simulink model "G431Hallcorrection"  (R2024a)
settings: Solver=FixedStepAuto  StartTime=0.0  StopTime=inf  RelTol=1e-3  EnableMultiTasking=on
undefined symbols (not defined in the file): DiscIntNeverNeededParam
libraries: stm32f4xxblockslib x11, mcbcontrolslib x7, simulink x6, mcbpositiondecoderlib x4, stm32g4xxblockslib x3, stm32blockslib x3, mcbsensorlessestimatorlib x2
settings Model: Creator=wsl  LastModifiedBy=wsl
settings SolverCC: AutoInsertRateTranBlk=on
settings DataIOCC: ReturnWorkspaceOutputs=off
settings OptimizationCC: EnhancedBackFolding=on  PassReuseOutputArgsAs=Individual arguments  ZeroExternalMemoryAtStartup=off  ZeroInternalMemoryAtStartup=off  MaxStackSize=64  OptimizeBlockOrder=speed  DifferentSizesBufferReuse=on  OptimizationCustomize=off  EfficientTunableParamExpr=on
settings DebuggingCC: MultiTaskDSMMsg=none  TasksWithSamePriorityMsg=none  ParameterPrecisionLossMsg=none  ParameterTunabilityLossMsg=error
settings HardwareCC: ProdBitPerPointer=32  ProdBitPerSizeT=32  ProdBitPerPtrDiffT=32  ProdLargestAtomicInteger=Long  ProdLargestAtomicFloat=Double  ProdWordSize=32  ProdLongLongMode=on  ProdHWDeviceType=ARM Compatible->ARM Cortex-M
settings SFSimCC: MATLABDynamicMemAlloc=off
settings RTWCC: Description=Embedded Coder  SystemTargetFile=ert.tlc  HardwareBoard=STM32G4xx Based  TemplateMakefile=ert_default_tmf  Toolchain=GNU Tools for ARM Embedded Processors
settings CodeAppCC: ForceParamTrailComments=on  IgnoreCustomStorageClasses=off  OperatorAnnotations=on  SimulinkDataObjDesc=on  SFDataObjDesc=on  InsertBlockDesc=on
settings ERTTargetCC: TargetLangStandard=C99 (ISO)  CodeReplacementLibrary=ARM Cortex-M  ExtModeTransport=3  ExtModeStaticAlloc=on  ExtModeStaticAllocSize=2048  ExtModeMexFile=ext_xcp  ExtModeIntrfLevel=Level2 - Open

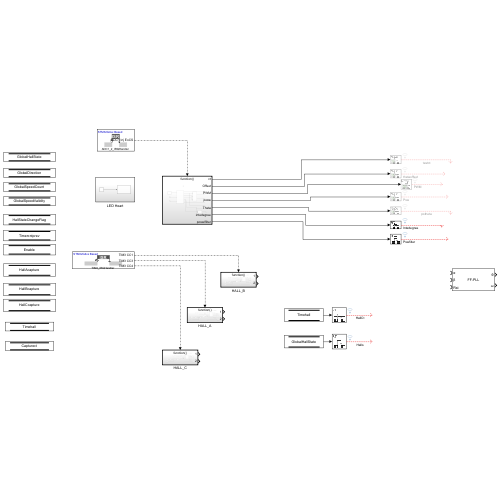
[thumbnail: Simulink's stored preview of the top-level diagram]
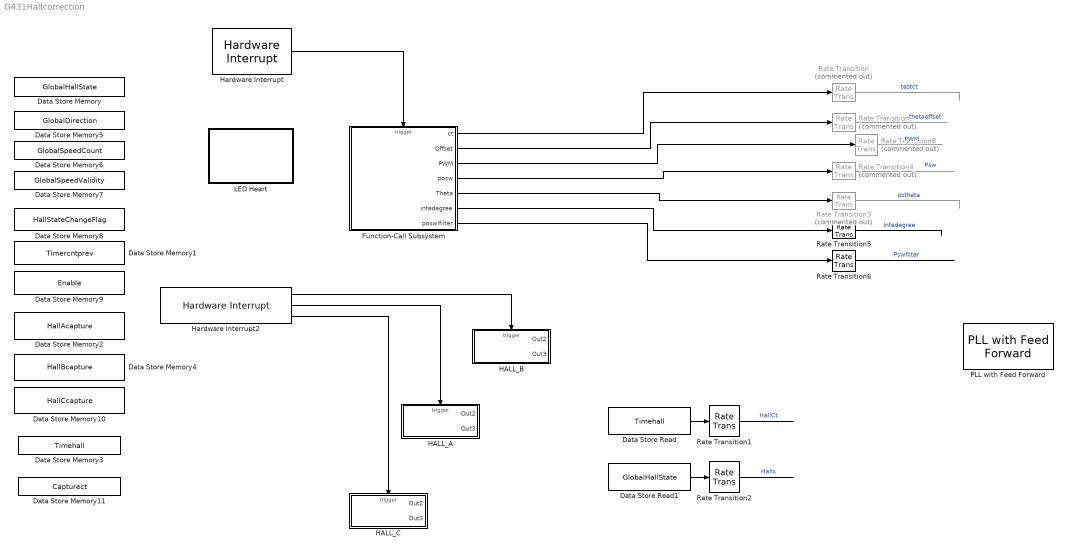
== system G431Hallcorrection ==
  Data Store Memory : DataStoreMemory  DataStoreName=GlobalHallState  WriteAfterWriteMsg=warning  ShowAdditionalParam=off
  Data Store Memory1 : DataStoreMemory  DataStoreName=Timercntprev  WriteAfterWriteMsg=warning  ShowAdditionalParam=off
  Data Store Memory10 : DataStoreMemory  DataStoreName=HallCcapture  WriteAfterWriteMsg=warning  ShowAdditionalParam=off
  Data Store Memory11 : DataStoreMemory  DataStoreName=Capturect  WriteAfterWriteMsg=warning  ShowAdditionalParam=off
  Data Store Memory2 : DataStoreMemory  DataStoreName=HallAcapture  WriteAfterWriteMsg=warning  ShowAdditionalParam=off
  Data Store Memory3 : DataStoreMemory  DataStoreName=Timehall  WriteAfterWriteMsg=warning  ShowAdditionalParam=off
  Data Store Memory4 : DataStoreMemory  DataStoreName=HallBcapture  WriteAfterWriteMsg=warning  ShowAdditionalParam=off
  Data Store Memory5 : DataStoreMemory  DataStoreName=GlobalDirection  WriteAfterWriteMsg=warning  ShowAdditionalParam=off
  Data Store Memory6 : DataStoreMemory  DataStoreName=GlobalSpeedCount  WriteAfterWriteMsg=warning  ShowAdditionalParam=off
  Data Store Memory7 : DataStoreMemory  DataStoreName=GlobalSpeedValidity  WriteAfterWriteMsg=warning  ShowAdditionalParam=off
  Data Store Memory8 : DataStoreMemory  DataStoreName=HallStateChangeFlag  WriteAfterWriteMsg=warning  ShowAdditionalParam=off
  Data Store Memory9 : DataStoreMemory  DataStoreName=Enable  WriteAfterWriteMsg=warning  ShowAdditionalParam=off
  Data Store Read : DataStoreRead  DataStoreName=Timehall  IndexOptions=Index vector (dialog)  Indices=1  OutputSizes=1
  Data Store Read1 : DataStoreRead  DataStoreName=GlobalHallState  IndexOptions=Index vector (dialog)  Indices=1  OutputSizes=1
  Function-Call Subsystem : Subsystem  TreatAsAtomicUnit=on
  HALL_A : Subsystem  TreatAsAtomicUnit=on
  HALL_B : Subsystem  TreatAsAtomicUnit=on
  HALL_C : Subsystem  TreatAsAtomicUnit=on
  Hardware Interrupt : stm32g4xxblockslib/Hardware Interrupt  ISRGroup=Analog to digital converter (ADC)  ISRName=ADC1_2_IRQHandler  ISRNumber=33  EventsList={ 'off', 'ADC1 OVR', '1'; 'off', 'ADC1 Reg EoCS', '2'; 'on', 'ADC1 Inj EoCS', '3'; 'off', 'ADC1 Inj JQOVF', '4'; 'off', 'ADC1 Watchdog1', '5'; 'off', 'ADC1 Watchdog2', '6'; 'off', 'ADC1 Watchdog3', '7'; 'off', 'ADC2 OVR', '8'; 'off', 'ADC2 Reg EoCS', '9'; 'off', 'ADC2 Inj EoCS', '10'; 'off', 'ADC2 Inj JQOVF', '11'; 'off', 'ADC2 Watchdog', '12'; 'off', 'ADC2 Watchdog2', '13'; 'off', 'ADC2 Watchdog3', '14'; 'off', 'Custom event', '15' }  SelectedEvents={'ADC1 Inj EoCS'}  TaskPriority=30  DisablePreemption=on  ClearInterruptFlagsAtEndOfEvent=off  InterruptDefinitionFile=$(TARGET_ROOT)/registry/interrupts/STM32F4xxBased_interrupts.xml  HardwareBoard=STM32G4xx Based  EnableSimPort=off
  Hardware Interrupt2 : stm32g4xxblockslib/Hardware Interrupt  ISRGroup=Timer (TIM)  ISRName=TIM3_IRQHandler  ISRNumber=44  EventsList={ 'off', 'TIM3 Update', '1'; 'on', 'TIM3 CC1', '2'; 'off', 'TIM3 CC2', '3'; 'on', 'TIM3 CC3', '4'; 'on', 'TIM3 CC4', '5'; 'off', 'TIM3 Trigger', '6'; 'off', 'TIM3 DIR', '7'; 'off', 'TIM3 IDX', '8'; 'off', 'TIM3 IERR', '9'; 'off', 'TIM3 TERR', '10'; 'off', 'Custom event', '11' }  SelectedEvents={'TIM3 CC1','TIM3 CC3','TIM3 CC4'}  TaskPriority=29  DisablePreemption=on  ClearInterruptFlagsAtEndOfEvent=off  InterruptDefinitionFile=$(TARGET_ROOT)/registry/interrupts/STM32F4xxBased_interrupts.xml  HardwareBoard=STM32G4xx Based  EnableSimPort=off
  LED Heart : Subsystem
  PLL with Feed Forward : mcbsensorlessestimatorlib/PLL with Feed Forward  Normalization=on  PosOut=Angular position  BlkSampleTime=50e-6  FreqRatio=1  MaximumApplicationFreq=7500  SpeedCutoffFreq=15  N_points=1024  Kp=942.4778  Ki=222066.099  PositionUnit=Degrees  PositionDataType=single  FrequencyUnit=Degrees/Sec  FrequencyDataType=single  TableDataType=single
      settings: LibrarySourceBlock=mcblib/Signal Management/PLL with Feed Forward
  Rate Transition{,3..4,7..8} (5 alike) : RateTransition  Commented=on  Integrity=off  OutPortSampleTime=1e-3
  Rate Transition{1..2,5..6} (4 alike) : RateTransition  Integrity=off  OutPortSampleTime=1e-3
  wires:
  Hardware Interrupt/1 -> Function-Call Subsystem/Trigger
  Function-Call Subsystem/1(ct) -> Rate Transition/1
  Rate Transition/1 -> ?  "testct"
  Data Store Read/1 -> Rate Transition1/1
  Rate Transition1/1 -> ?  "HallCt"
  Hardware Interrupt2/3 -> HALL_C/Trigger
  Hardware Interrupt2/1 -> HALL_B/Trigger
  Hardware Interrupt2/2 -> HALL_A/Trigger
  Rate Transition2/1 -> ?  "Halls"
  Data Store Read1/1 -> Rate Transition2/1
  Rate Transition3/1 -> ?  "pstheta"
  Function-Call Subsystem/5(Theta) -> Rate Transition3/1
  Rate Transition4/1 -> ?  "Psw"
  Function-Call Subsystem/6(intedegree) -> Rate Transition5/1
  Rate Transition5/1 -> ?  "Intedegree"
  Function-Call Subsystem/4(posw) -> Rate Transition4/1
  Rate Transition6/1 -> ?  "Pswfilter"
  Function-Call Subsystem/7(poswlfilter) -> Rate Transition6/1
  Function-Call Subsystem/2(Offset) -> Rate Transition7/1
  Rate Transition7/1 -> ?  "thetaoffset"
  Function-Call Subsystem/3(PWM) -> Rate Transition8/1
  Rate Transition8/1 -> ?  "PWM"

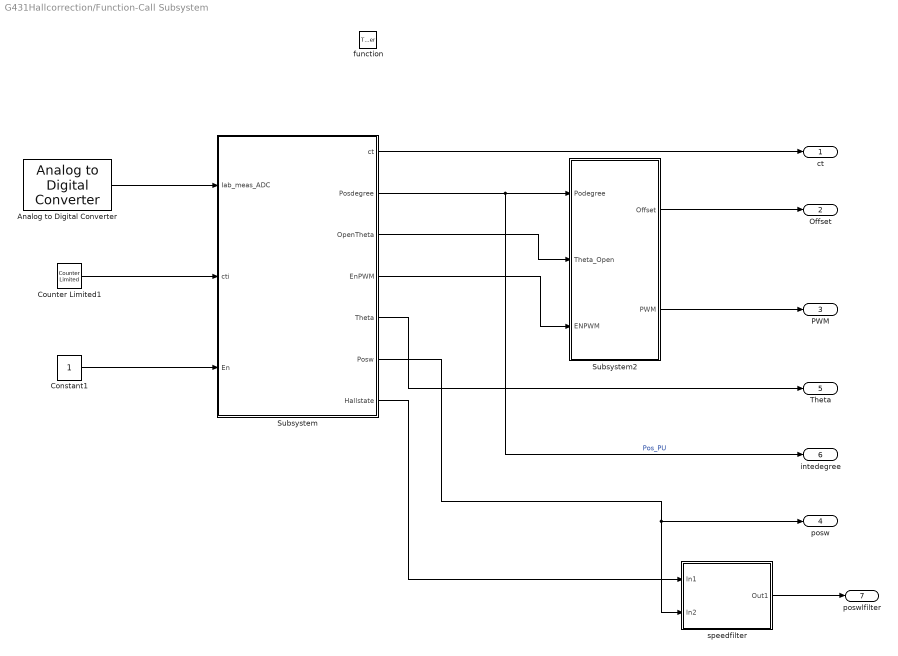
== system G431Hallcorrection/Function-Call Subsystem ==
  function : TriggerPort  TriggerType=function-call  VariantControl=(inherit)
  Analog to Digital Converter : stm32f4xxblockslib/Analog to Digital Converter  ADCModule=ADC1  ConversionGroup=Injected  TriggerMode=Read results only  NumberOfConversions=3  EnableBufferConv=off  BufferLength=1  OutputStatus=off  SampleTime=-1  EnableSimPort=off
  Constant1 : Constant  VectorParams1D=off
  Counter Limited1 : simulink/Sources/Counter Limited  uplimit=20000  tsamp=-1
  Subsystem : Subsystem
  Subsystem2 : Subsystem
  "speedfilter " : Subsystem
  ct : Outport
  Offset : Outport  Port=2
  PWM : Outport  Port=3
  posw : Outport  Port=4
  Theta : Outport  Port=5
  intedegree : Outport  Port=6
  poswlfilter : Outport  Port=7
  wires:
  Analog to Digital Converter/1 -> Subsystem/1(Iab_meas_ADC)
  Subsystem/4(EnPWM) -> Subsystem2/3(ENPWM)
  Subsystem2/2(PWM) -> PWM/1
  Constant1/1 -> Subsystem/3(En)
  Subsystem/1(ct) -> ct/1
  Subsystem2/1(Offset) -> Offset/1
  Subsystem/2(Posdegree) -> intedegree/1, Subsystem2/1(Podegree)  "Pos_PU"
  Counter Limited1/1 -> Subsystem/2(cti)
  Subsystem/3(OpenTheta) -> Subsystem2/2(Theta_Open)
  Subsystem/5(Theta) -> Theta/1
  Subsystem/6(Posw) -> "speedfilter "/2(In2), posw/1
  Subsystem/7(Hallstate) -> "speedfilter "/1(In1)
  "speedfilter "/1(Out1) -> poswlfilter/1

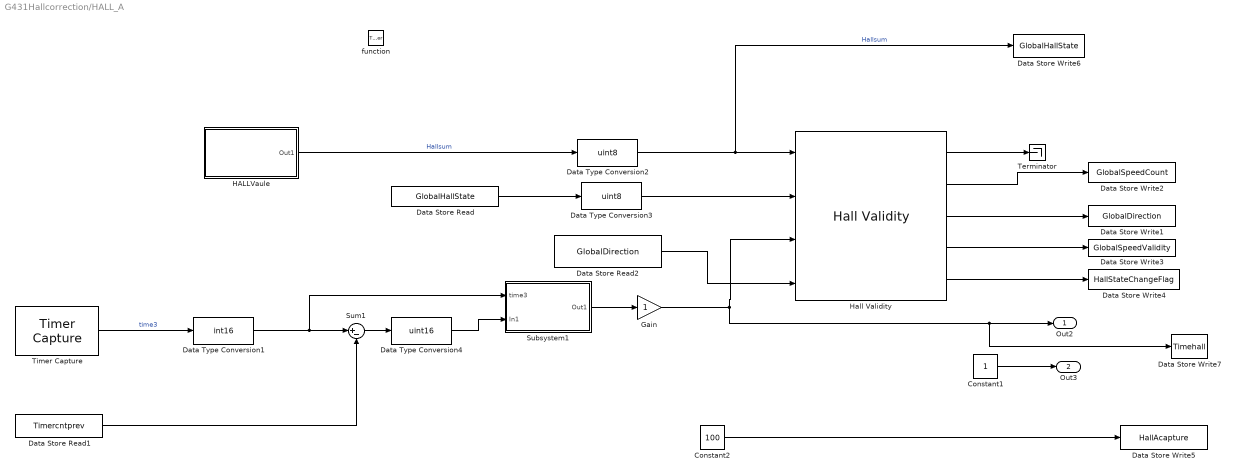
== system G431Hallcorrection/HALL_A ==
  function : TriggerPort  TriggerType=function-call  VariantControl=(inherit)
  Constant1 : Constant
  Constant2 : Constant  Value=100
  Data Store Read : DataStoreRead  DataStoreName=GlobalHallState  IndexOptions=Index vector (dialog)  Indices=1  OutputSizes=1
  Data Store Read1 : DataStoreRead  DataStoreName=Timercntprev  IndexOptions=Index vector (dialog)  Indices=1  OutputSizes=1
  Data Store Read2 : DataStoreRead  DataStoreName=GlobalDirection  IndexOptions=Index vector (dialog)  Indices=1  OutputSizes=1
  Data Store Write1 : DataStoreWrite  DataStoreName=GlobalDirection  IndexOptions=Index vector (dialog)  Indices=1  OutputSizes=1
  Data Store Write2 : DataStoreWrite  DataStoreName=GlobalSpeedCount  IndexOptions=Index vector (dialog)  Indices=1  OutputSizes=1
  Data Store Write3 : DataStoreWrite  DataStoreName=GlobalSpeedValidity  IndexOptions=Index vector (dialog)  Indices=1  OutputSizes=1
  Data Store Write4 : DataStoreWrite  DataStoreName=HallStateChangeFlag  IndexOptions=Index vector (dialog)  Indices=1  OutputSizes=1
  Data Store Write5 : DataStoreWrite  DataStoreName=HallAcapture  IndexOptions=Index vector (dialog)  Indices=1  OutputSizes=1
  Data Store Write6 : DataStoreWrite  DataStoreName=GlobalHallState  IndexOptions=Index vector (dialog)  Indices=1  OutputSizes=1
  Data Store Write7 : DataStoreWrite  DataStoreName=Timehall  IndexOptions=Index vector (dialog)  Indices=1  OutputSizes=1
  Data Type Conversion1 : DataTypeConversion  OutDataTypeStr=int16  SaturateOnIntegerOverflow=off  RndMeth=Floor
  Data Type Conversion2 : DataTypeConversion  OutDataTypeStr=uint8  SaturateOnIntegerOverflow=off  RndMeth=Floor
  Data Type Conversion3 : DataTypeConversion  OutDataTypeStr=uint8  SaturateOnIntegerOverflow=off  RndMeth=Floor
  Data Type Conversion4 : DataTypeConversion  OutDataTypeStr=uint16  SaturateOnIntegerOverflow=off  RndMeth=Floor
  Gain : Gain
  HALLVaule : Subsystem
  Hall Validity : mcbpositiondecoderlib/Hall Validity  hallSequence=ABC  sequence=[5,4,6,2,3,1]  CounterSize=16 bits
  Subsystem1 : Subsystem
  Sum1 : Sum  Inputs=|+-
  Terminator : Terminator
  Timer Capture : stm32blockslib/Timer Capture  TimerModule=TIM3  SelectedChannel=CH3  CaptureLength=1  OutputDataLength=off  OutputOverrunStatus=off  OutputDirection=off  SampleTime=-1
      settings: LibrarySourceBlock=stm32g4xxblockslib/Timer Capture
  Out2 : Outport
  Out3 : Outport  Port=2
  wires:
  Hall Validity/4 -> Data Store Write3/1
  HALLVaule/1(Out1) -> Data Type Conversion2/1  "Hallsum"
  Data Type Conversion3/1 -> Hall Validity/2
  Data Store Read2/1 -> Hall Validity/4
  Gain/1 -> Data Store Write7/1, Out2/1, Hall Validity/3
  Data Type Conversion2/1 -> Data Store Write6/1, Hall Validity/1  "Hallsum"
  Hall Validity/3 -> Data Store Write1/1
  Constant1/1 -> Out3/1
  Hall Validity/2 -> Data Store Write2/1
  Hall Validity/1 -> Terminator/1
  Constant2/1 -> Data Store Write5/1
  Hall Validity/5 -> Data Store Write4/1
  Data Store Read/1 -> Data Type Conversion3/1
  Sum1/1 -> Data Type Conversion4/1
  Data Store Read1/1 -> Sum1/2
  Data Type Conversion1/1 -> Sum1/1, Subsystem1/1(time3)
  Timer Capture/1 -> Data Type Conversion1/1  "time3"
  Data Type Conversion4/1 -> Subsystem1/2(In1)
  Subsystem1/1(Out1) -> Gain/1

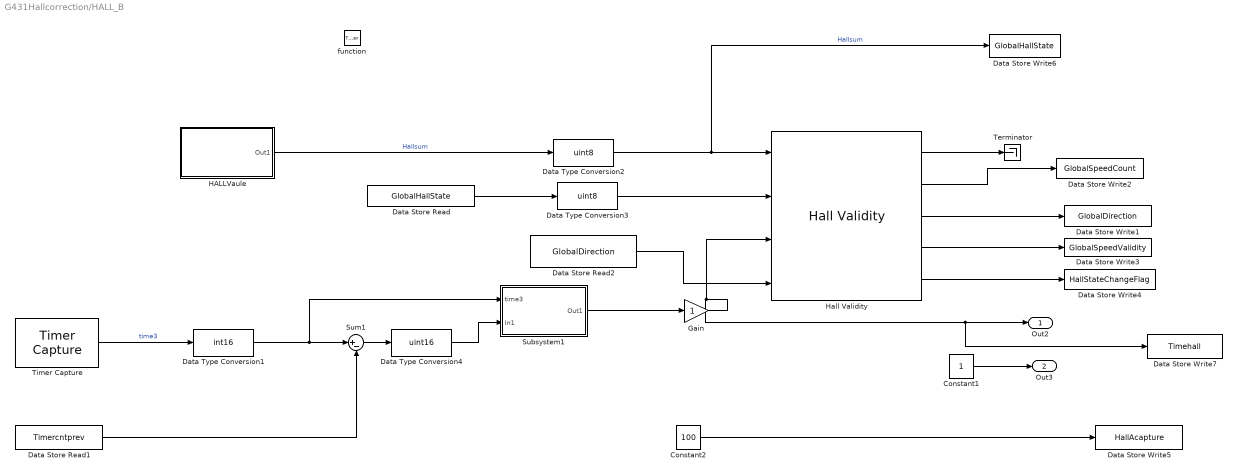
== system G431Hallcorrection/HALL_B ==
  function : TriggerPort  TriggerType=function-call  VariantControl=(inherit)
  Constant1 : Constant
  Constant2 : Constant  Value=100
  Data Store Read : DataStoreRead  DataStoreName=GlobalHallState  IndexOptions=Index vector (dialog)  Indices=1  OutputSizes=1
  Data Store Read1 : DataStoreRead  DataStoreName=Timercntprev  IndexOptions=Index vector (dialog)  Indices=1  OutputSizes=1
  Data Store Read2 : DataStoreRead  DataStoreName=GlobalDirection  IndexOptions=Index vector (dialog)  Indices=1  OutputSizes=1
  Data Store Write1 : DataStoreWrite  DataStoreName=GlobalDirection  IndexOptions=Index vector (dialog)  Indices=1  OutputSizes=1
  Data Store Write2 : DataStoreWrite  DataStoreName=GlobalSpeedCount  IndexOptions=Index vector (dialog)  Indices=1  OutputSizes=1
  Data Store Write3 : DataStoreWrite  DataStoreName=GlobalSpeedValidity  IndexOptions=Index vector (dialog)  Indices=1  OutputSizes=1
  Data Store Write4 : DataStoreWrite  DataStoreName=HallStateChangeFlag  IndexOptions=Index vector (dialog)  Indices=1  OutputSizes=1
  Data Store Write5 : DataStoreWrite  DataStoreName=HallAcapture  IndexOptions=Index vector (dialog)  Indices=1  OutputSizes=1
  Data Store Write6 : DataStoreWrite  DataStoreName=GlobalHallState  IndexOptions=Index vector (dialog)  Indices=1  OutputSizes=1
  Data Store Write7 : DataStoreWrite  DataStoreName=Timehall  IndexOptions=Index vector (dialog)  Indices=1  OutputSizes=1
  Data Type Conversion1 : DataTypeConversion  OutDataTypeStr=int16  SaturateOnIntegerOverflow=off  RndMeth=Floor
  Data Type Conversion2 : DataTypeConversion  OutDataTypeStr=uint8  SaturateOnIntegerOverflow=off  RndMeth=Floor
  Data Type Conversion3 : DataTypeConversion  OutDataTypeStr=uint8  SaturateOnIntegerOverflow=off  RndMeth=Floor
  Data Type Conversion4 : DataTypeConversion  OutDataTypeStr=uint16  SaturateOnIntegerOverflow=off  RndMeth=Floor
  Gain : Gain
  HALLVaule : Subsystem
  Hall Validity : mcbpositiondecoderlib/Hall Validity  hallSequence=ABC  sequence=[5,4,6,2,3,1]  CounterSize=16 bits
  Subsystem1 : Subsystem
  Sum1 : Sum  Inputs=|+-
  Terminator : Terminator
  Timer Capture : stm32blockslib/Timer Capture  TimerModule=TIM3  SelectedChannel=CH1  CaptureLength=1  OutputDataLength=off  OutputOverrunStatus=off  OutputDirection=off  SampleTime=-1
      settings: LibrarySourceBlock=stm32g4xxblockslib/Timer Capture
  Out2 : Outport
  Out3 : Outport  Port=2
  wires:
  Hall Validity/4 -> Data Store Write3/1
  HALLVaule/1(Out1) -> Data Type Conversion2/1  "Hallsum"
  Data Type Conversion3/1 -> Hall Validity/2
  Data Store Read2/1 -> Hall Validity/4
  Gain/1 -> Data Store Write7/1, Out2/1, Hall Validity/3
  Data Type Conversion2/1 -> Data Store Write6/1, Hall Validity/1  "Hallsum"
  Hall Validity/3 -> Data Store Write1/1
  Constant1/1 -> Out3/1
  Hall Validity/1 -> Terminator/1
  Constant2/1 -> Data Store Write5/1
  Hall Validity/5 -> Data Store Write4/1
  Data Store Read/1 -> Data Type Conversion3/1
  Data Type Conversion4/1 -> Subsystem1/2(In1)
  Sum1/1 -> Data Type Conversion4/1
  Timer Capture/1 -> Data Type Conversion1/1  "time3"
  Data Type Conversion1/1 -> Sum1/1, Subsystem1/1(time3)
  Data Store Read1/1 -> Sum1/2
  Subsystem1/1(Out1) -> Gain/1
  Hall Validity/2 -> Data Store Write2/1

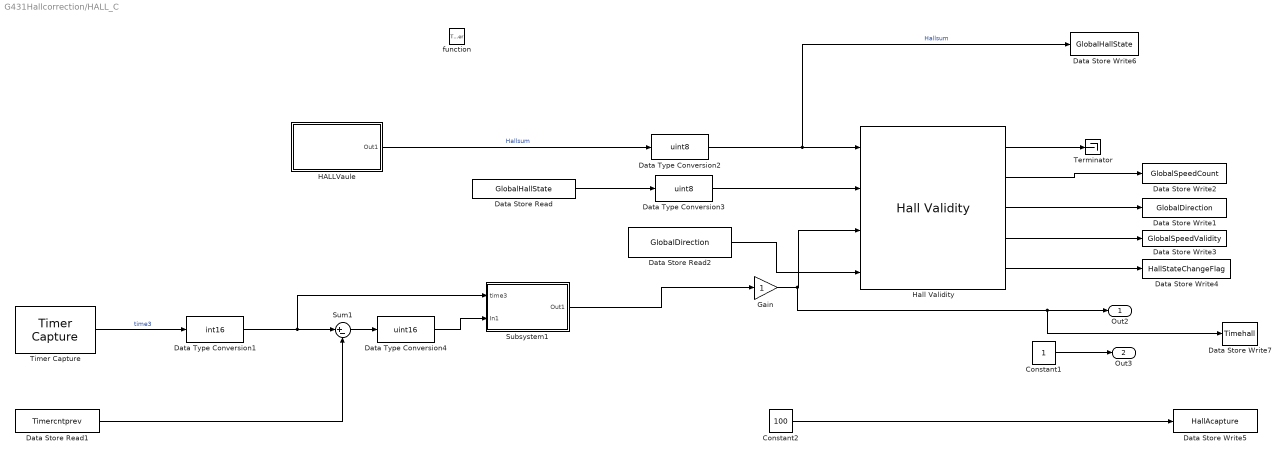
== system G431Hallcorrection/HALL_C ==
  function : TriggerPort  TriggerType=function-call  VariantControl=(inherit)
  Constant1 : Constant
  Constant2 : Constant  Value=100
  Data Store Read : DataStoreRead  DataStoreName=GlobalHallState  IndexOptions=Index vector (dialog)  Indices=1  OutputSizes=1
  Data Store Read1 : DataStoreRead  DataStoreName=Timercntprev  IndexOptions=Index vector (dialog)  Indices=1  OutputSizes=1
  Data Store Read2 : DataStoreRead  DataStoreName=GlobalDirection  IndexOptions=Index vector (dialog)  Indices=1  OutputSizes=1
  Data Store Write1 : DataStoreWrite  DataStoreName=GlobalDirection  IndexOptions=Index vector (dialog)  Indices=1  OutputSizes=1
  Data Store Write2 : DataStoreWrite  DataStoreName=GlobalSpeedCount  IndexOptions=Index vector (dialog)  Indices=1  OutputSizes=1
  Data Store Write3 : DataStoreWrite  DataStoreName=GlobalSpeedValidity  IndexOptions=Index vector (dialog)  Indices=1  OutputSizes=1
  Data Store Write4 : DataStoreWrite  DataStoreName=HallStateChangeFlag  IndexOptions=Index vector (dialog)  Indices=1  OutputSizes=1
  Data Store Write5 : DataStoreWrite  DataStoreName=HallAcapture  IndexOptions=Index vector (dialog)  Indices=1  OutputSizes=1
  Data Store Write6 : DataStoreWrite  DataStoreName=GlobalHallState  IndexOptions=Index vector (dialog)  Indices=1  OutputSizes=1
  Data Store Write7 : DataStoreWrite  DataStoreName=Timehall  IndexOptions=Index vector (dialog)  Indices=1  OutputSizes=1
  Data Type Conversion1 : DataTypeConversion  OutDataTypeStr=int16  SaturateOnIntegerOverflow=off  RndMeth=Floor
  Data Type Conversion2 : DataTypeConversion  OutDataTypeStr=uint8  SaturateOnIntegerOverflow=off  RndMeth=Floor
  Data Type Conversion3 : DataTypeConversion  OutDataTypeStr=uint8  SaturateOnIntegerOverflow=off  RndMeth=Floor
  Data Type Conversion4 : DataTypeConversion  OutDataTypeStr=uint16  SaturateOnIntegerOverflow=off  RndMeth=Floor
  Gain : Gain
  HALLVaule : Subsystem
  Hall Validity : mcbpositiondecoderlib/Hall Validity  hallSequence=ABC  sequence=[5,4,6,2,3,1]  CounterSize=16 bits
  Subsystem1 : Subsystem
  Sum1 : Sum  Inputs=|+-
  Terminator : Terminator
  Timer Capture : stm32blockslib/Timer Capture  TimerModule=TIM3  SelectedChannel=CH4  CaptureLength=1  OutputDataLength=off  OutputOverrunStatus=off  OutputDirection=off  SampleTime=-1
      settings: LibrarySourceBlock=stm32g4xxblockslib/Timer Capture
  Out2 : Outport
  Out3 : Outport  Port=2
  wires:
  Hall Validity/4 -> Data Store Write3/1
  HALLVaule/1(Out1) -> Data Type Conversion2/1  "Hallsum"
  Data Type Conversion3/1 -> Hall Validity/2
  Data Store Read2/1 -> Hall Validity/4
  Gain/1 -> Data Store Write7/1, Out2/1, Hall Validity/3
  Data Type Conversion2/1 -> Data Store Write6/1, Hall Validity/1  "Hallsum"
  Hall Validity/3 -> Data Store Write1/1
  Constant1/1 -> Out3/1
  Hall Validity/1 -> Terminator/1
  Constant2/1 -> Data Store Write5/1
  Hall Validity/5 -> Data Store Write4/1
  Data Store Read/1 -> Data Type Conversion3/1
  Data Type Conversion4/1 -> Subsystem1/2(In1)
  Sum1/1 -> Data Type Conversion4/1
  Timer Capture/1 -> Data Type Conversion1/1  "time3"
  Data Type Conversion1/1 -> Sum1/1, Subsystem1/1(time3)
  Data Store Read1/1 -> Sum1/2
  Subsystem1/1(Out1) -> Gain/1
  Hall Validity/2 -> Data Store Write2/1

== system G431Hallcorrection/LED Heart ==
  Digital Port Write : stm32f4xxblockslib/Digital Port Write  PortName=GPIOA  PinNumber=[5]  ReadOperation=off  IOAsArray=on  EnableSimPort=off
      settings: LibrarySourceBlock=stm32g4xxblockslib/Digital Port Write
  Pulse Generator : DiscretePulseGenerator  Period=10  PulseWidth=5  SampleTime=0.1
  wires:
  Pulse Generator/1 -> Digital Port Write/1  "LED"

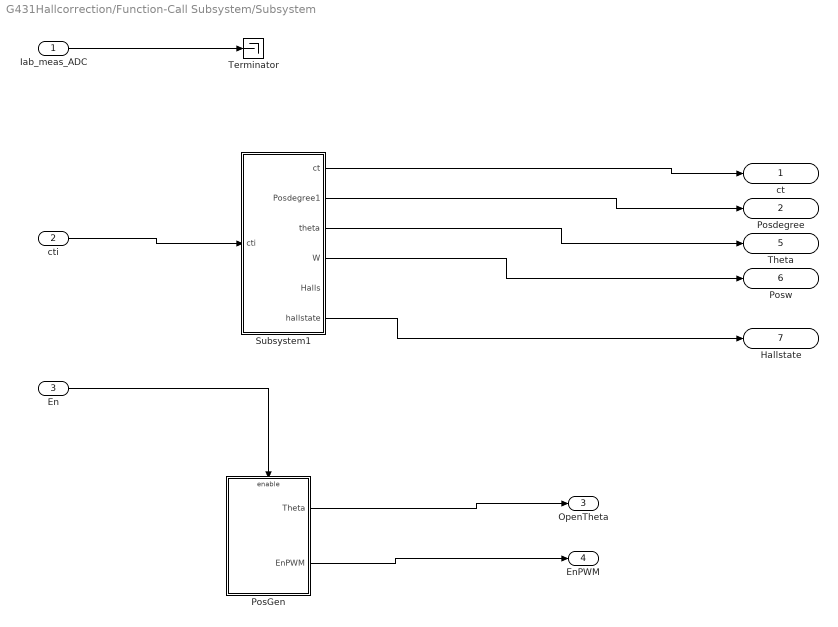
== system G431Hallcorrection/Function-Call Subsystem/Subsystem ==
  Iab_meas_ADC : Inport  OutDataTypeStr=uint16
  cti : Inport  Port=2
  En : Inport  Port=3
  PosGen : Subsystem
  Subsystem1 : Subsystem
  Terminator : Terminator
  ct : Outport
  Posdegree : Outport  Port=2
  OpenTheta : Outport  Port=3
  EnPWM : Outport  Port=4
  Theta : Outport  Port=5
  Posw : Outport  Port=6
  Hallstate : Outport  Port=7
  wires:
  Iab_meas_ADC/1 -> Terminator/1
  Subsystem1/2(Posdegree1) -> Posdegree/1
  Subsystem1/1(ct) -> ct/1
  cti/1 -> Subsystem1/1(cti)
  PosGen/1(Theta) -> OpenTheta/1
  PosGen/2(EnPWM) -> EnPWM/1
  En/1 -> PosGen/Enable
  Subsystem1/3(theta) -> Theta/1
  Subsystem1/4(W) -> Posw/1
  Subsystem1/6(hallstate) -> Hallstate/1

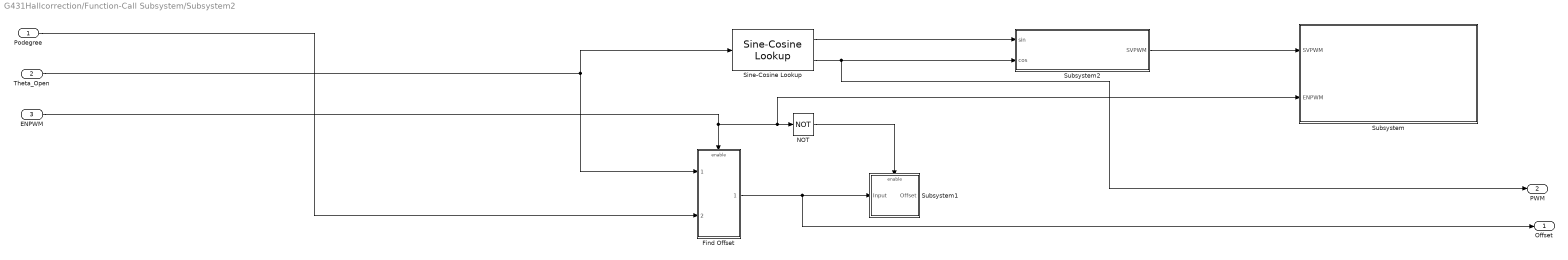
== system G431Hallcorrection/Function-Call Subsystem/Subsystem2 ==
  Podegree : Inport
  Theta_Open : Inport  Port=2
  ENPWM : Inport  Port=3
  Find Offset : Subsystem
  NOT : Logic  Operator=NOT  IconShape=distinctive  AllPortsSameDT=off  OutDataTypeStr=boolean
  Sine-Cosine Lookup : mcbcontrolslib/Sine-Cosine Lookup  AngleInput=Per-unit  N_points=1024  DatatypeInput=Inherit from input  Datatype=single
  Subsystem : Subsystem
  Subsystem1 : Subsystem
  Subsystem2 : Subsystem
  Offset : Outport
  PWM : Outport  Port=2
  wires:
  ENPWM/1 -> Subsystem/2(ENPWM), NOT/1, Find Offset/Enable
  Podegree/1 -> Find Offset/2(Theta_hall)
  Theta_Open/1 -> Sine-Cosine Lookup/1, Find Offset/1(Theta_Open)
  Sine-Cosine Lookup/2 -> Subsystem2/2(cos), PWM/1
  Find Offset/1(Offset) -> Offset/1, Subsystem1/1(Input)
  NOT/1 -> Subsystem1/Enable
  Sine-Cosine Lookup/1 -> Subsystem2/1(sin)
  Subsystem2/1("SVPWM ") -> Subsystem/1(SVPWM)

== system G431Hallcorrection/Function-Call Subsystem/speedfilter  ==
  In1 : Inport
  In2 : Inport  Port=2
  Compare speed low than 20RPM : simulink/Logic and Bit Operations/Compare To Constant  relop=<=  const=120  OutDataTypeStr=boolean
  Enabled Subsystem : Subsystem  TreatAsAtomicUnit=on
  IIR Filter : mcbcontrolslib/IIR Filter  VariantControl=Low Pass Filter  VariantSelect=Low-pass  FilterConstantInputType=Specify via dialog  Filter_constant=0.001  advancedSettings=on  Ts=1e-4  cutOff_freq=1.5931
      settings: LibrarySourceBlock=mcbhdllib/Signal Management/IIR Filter
  IIR Filter1 : mcbcontrolslib/IIR Filter  VariantControl=Low Pass Filter  VariantSelect=Low-pass  FilterConstantInputType=Specify via dialog  Filter_constant=0.003  advancedSettings=on  Ts=1e-4  cutOff_freq=4.789
      settings: LibrarySourceBlock=mcbhdllib/Signal Management/IIR Filter
  OR : Logic  Operator=OR  IconShape=distinctive  AllPortsSameDT=off  OutDataTypeStr=boolean
  Out1 : Outport
  wires:
  Enabled Subsystem/1(poswlfilter) -> IIR Filter/1
  IIR Filter1/1 -> Compare speed low than 20RPM/1, Enabled Subsystem/1(In1)
  In2/1 -> IIR Filter1/1
  IIR Filter/1 -> Out1/1
  OR/1 -> Enabled Subsystem/Enable
  Compare speed low than 20RPM/1 -> OR/2
  In1/1 -> OR/1

== system G431Hallcorrection/HALL_A/HALLVaule ==
  Gain : Gain  Gain=4
  Gain1 : Gain  Gain=2
  HALLB : stm32f4xxblockslib/Digital Port Read  PortName=GPIOC  PinNumber=[6]  ReadOperation=on  IOAsArray=on  SampleTime=-1  EnableSimPort=off
      settings: LibrarySourceBlock=stm32g4xxblockslib/Digital Port Read
  HALLB1 : stm32f4xxblockslib/Digital Port Read  PortName=GPIOC  PinNumber=[8]  ReadOperation=on  IOAsArray=on  SampleTime=-1  EnableSimPort=off
      settings: LibrarySourceBlock=stm32g4xxblockslib/Digital Port Read
  HALLC : stm32f4xxblockslib/Digital Port Read  PortName=GPIOC  PinNumber=[9]  ReadOperation=on  IOAsArray=on  SampleTime=-1  EnableSimPort=off
      settings: LibrarySourceBlock=stm32g4xxblockslib/Digital Port Read
  Sum : Sum  Inputs=|+++
  Out1 : Outport
  wires:
  HALLB/1 -> Gain1/1
  HALLB1/1 -> Gain/1
  Gain/1 -> Sum/1
  HALLC/1 -> Sum/3
  Gain1/1 -> Sum/2
  Sum/1 -> Out1/1

== system G431Hallcorrection/HALL_A/Subsystem1 ==
  time3 : Inport
  In1 : Inport  Port=2
  Data Store Write : DataStoreWrite  DataStoreName=Timercntprev  IndexOptions=Index vector (dialog)  Indices=1  OutputSizes=1
  Out1 : Outport
  wires:
  time3/1 -> Data Store Write/1
  In1/1 -> Out1/1

== system G431Hallcorrection/HALL_B/HALLVaule ==
  Gain : Gain  Gain=4
  Gain1 : Gain  Gain=2
  HALLB : stm32f4xxblockslib/Digital Port Read  PortName=GPIOC  PinNumber=[6]  ReadOperation=on  IOAsArray=on  SampleTime=-1  EnableSimPort=off
      settings: LibrarySourceBlock=stm32g4xxblockslib/Digital Port Read
  HALLB1 : stm32f4xxblockslib/Digital Port Read  PortName=GPIOC  PinNumber=[8]  ReadOperation=on  IOAsArray=on  SampleTime=-1  EnableSimPort=off
      settings: LibrarySourceBlock=stm32g4xxblockslib/Digital Port Read
  HALLC : stm32f4xxblockslib/Digital Port Read  PortName=GPIOC  PinNumber=[9]  ReadOperation=on  IOAsArray=on  SampleTime=-1  EnableSimPort=off
      settings: LibrarySourceBlock=stm32g4xxblockslib/Digital Port Read
  Sum : Sum  Inputs=|+++
  Out1 : Outport
  wires:
  HALLB/1 -> Gain1/1
  HALLB1/1 -> Gain/1
  Gain/1 -> Sum/1
  HALLC/1 -> Sum/3
  Gain1/1 -> Sum/2
  Sum/1 -> Out1/1

== system G431Hallcorrection/HALL_B/Subsystem1 ==
  time3 : Inport
  In1 : Inport  Port=2
  Data Store Write : DataStoreWrite  DataStoreName=Timercntprev  IndexOptions=Index vector (dialog)  Indices=1  OutputSizes=1
  Out1 : Outport
  wires:
  time3/1 -> Data Store Write/1
  In1/1 -> Out1/1

== system G431Hallcorrection/HALL_C/HALLVaule ==
  Gain : Gain  Gain=4
  Gain1 : Gain  Gain=2
  HALLB : stm32f4xxblockslib/Digital Port Read  PortName=GPIOC  PinNumber=[6]  ReadOperation=on  IOAsArray=on  SampleTime=-1  EnableSimPort=off
      settings: LibrarySourceBlock=stm32g4xxblockslib/Digital Port Read
  HALLB1 : stm32f4xxblockslib/Digital Port Read  PortName=GPIOC  PinNumber=[8]  ReadOperation=on  IOAsArray=on  SampleTime=-1  EnableSimPort=off
      settings: LibrarySourceBlock=stm32g4xxblockslib/Digital Port Read
  HALLC : stm32f4xxblockslib/Digital Port Read  PortName=GPIOC  PinNumber=[9]  ReadOperation=on  IOAsArray=on  SampleTime=-1  EnableSimPort=off
      settings: LibrarySourceBlock=stm32g4xxblockslib/Digital Port Read
  Sum : Sum  Inputs=|+++
  Out1 : Outport
  wires:
  HALLB/1 -> Gain1/1
  HALLB1/1 -> Gain/1
  Gain/1 -> Sum/1
  HALLC/1 -> Sum/3
  Gain1/1 -> Sum/2
  Sum/1 -> Out1/1

== system G431Hallcorrection/HALL_C/Subsystem1 ==
  time3 : Inport
  In1 : Inport  Port=2
  Data Store Write : DataStoreWrite  DataStoreName=Timercntprev  IndexOptions=Index vector (dialog)  Indices=1  OutputSizes=1
  Out1 : Outport
  wires:
  time3/1 -> Data Store Write/1
  In1/1 -> Out1/1

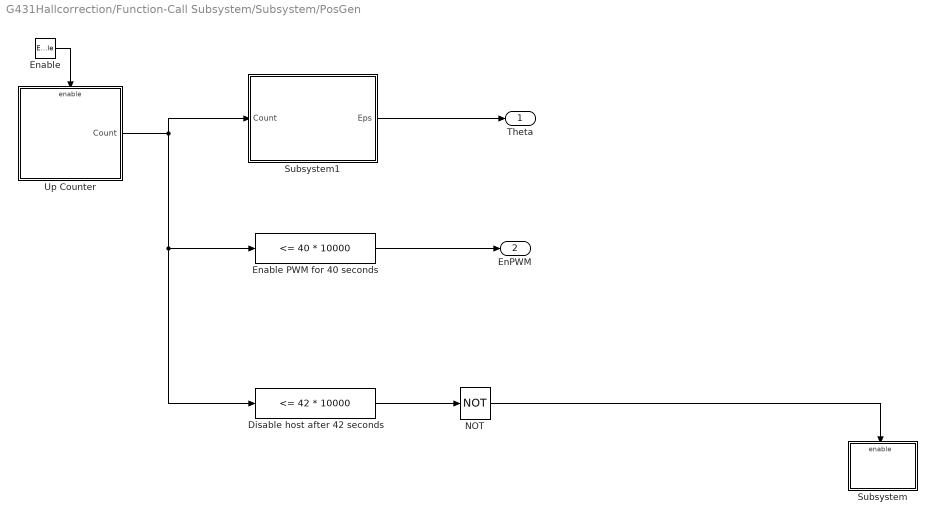
== system G431Hallcorrection/Function-Call Subsystem/Subsystem/PosGen ==
  Enable : EnablePort  StatesWhenEnabling=reset  ShowOutputPort=on
  Disable host after 42 seconds : simulink/Logic and Bit Operations/Compare To Constant  relop=<=  const=42 * 10000  OutDataTypeStr=boolean
  Enable PWM for 40 seconds : simulink/Logic and Bit Operations/Compare To Constant  relop=<=  const=40 * 10000  OutDataTypeStr=boolean
  NOT : Logic  Operator=NOT  IconShape=distinctive  AllPortsSameDT=off  OutDataTypeStr=boolean
  Subsystem : Subsystem
  Subsystem1 : Subsystem
  Up Counter : Subsystem
  Theta : Outport
  EnPWM : Outport  Port=2  OutputWhenDisabled=reset  InitialOutput=0  VectorParamsAs1DForOutWhenUnconnected=off
  wires:
  Subsystem1/1(Eps) -> Theta/1
  Up Counter/1(Count) -> Subsystem1/1(Count), Disable host after 42 seconds/1, Enable PWM for 40 seconds/1
  Enable/1 -> Up Counter/Enable
  NOT/1 -> Subsystem/Enable
  Enable PWM for 40 seconds/1 -> EnPWM/1
  Disable host after 42 seconds/1 -> NOT/1

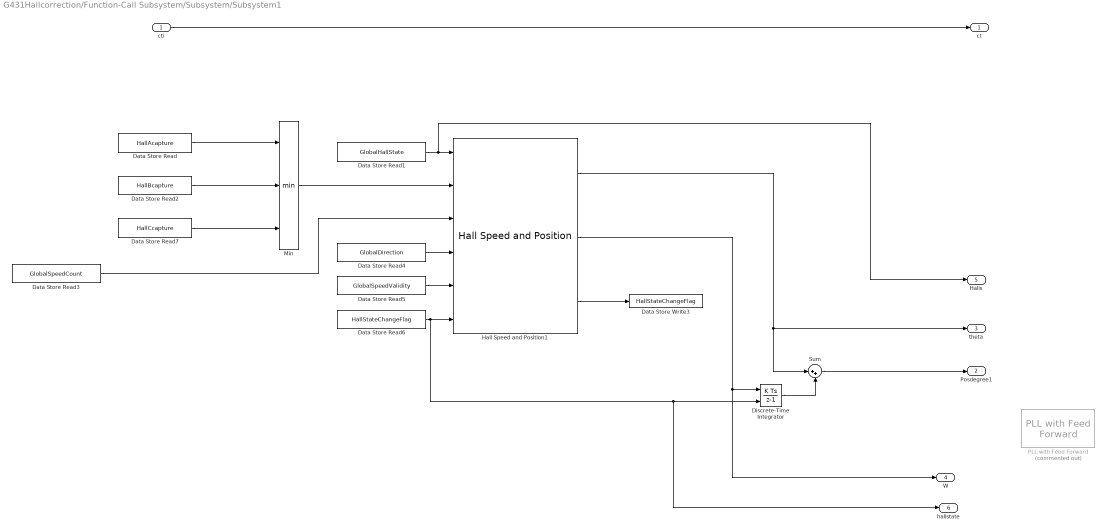
== system G431Hallcorrection/Function-Call Subsystem/Subsystem/Subsystem1 ==
  cti : Inport
  Data Store Read : DataStoreRead  DataStoreName=HallAcapture  IndexOptions=Index vector (dialog)  Indices=1  OutputSizes=1
  Data Store Read1 : DataStoreRead  DataStoreName=GlobalHallState  IndexOptions=Index vector (dialog)  Indices=1  OutputSizes=1
  Data Store Read2 : DataStoreRead  DataStoreName=HallBcapture  IndexOptions=Index vector (dialog)  Indices=1  OutputSizes=1
  Data Store Read3 : DataStoreRead  DataStoreName=GlobalSpeedCount  IndexOptions=Index vector (dialog)  Indices=1  OutputSizes=1
  Data Store Read4 : DataStoreRead  DataStoreName=GlobalDirection  IndexOptions=Index vector (dialog)  Indices=1  OutputSizes=1
  Data Store Read5 : DataStoreRead  DataStoreName=GlobalSpeedValidity  IndexOptions=Index vector (dialog)  Indices=1  OutputSizes=1
  Data Store Read6 : DataStoreRead  Priority=1  DataStoreName=HallStateChangeFlag  IndexOptions=Index vector (dialog)  Indices=1  OutputSizes=1
  Data Store Read7 : DataStoreRead  DataStoreName=HallCcapture  IndexOptions=Index vector (dialog)  Indices=1  OutputSizes=1
  Data Store Write3 : DataStoreWrite  Priority=2  DataStoreName=HallStateChangeFlag  IndexOptions=Index vector (dialog)  Indices=1  OutputSizes=1
  Discrete-Time Integrator : DiscreteIntegrator  ExternalReset=rising  SampleTime=-1  LimitOutput=on  UpperSaturationLimit=60  LowerSaturationLimit=-60  ICPrevOutput=DiscIntNeverNeededParam  ICPrevScaledInput=DiscIntNeverNeededParam
  Hall Speed and Position1 : mcbpositiondecoderlib/Hall Speed and Position  blkExecutionType=Speed and position  CounterSize=16 bits  ClkFreq=1e5  BlkSampleTime=1e-4  PolePairs=1  MinSpeed=20  HallInterruptConfig=Every 60 Degrees  SpeedUnit=Degrees/sec  PerUnitSpeed=60  SpeedDataType=single  hallSequence=ABC  Sequence=[5,4,6,2,3,1]  EnableSecondOrder=1st Order  PositionUnit=Degrees  PositionDataType=single
  Min : MinMax  Inputs=3
  PLL with Feed Forward : mcbsensorlessestimatorlib/PLL with Feed Forward  Commented=on  Normalization=on  PosOut=Angular position  BlkSampleTime=50e-6  FreqRatio=1  MaximumApplicationFreq=7500  SpeedCutoffFreq=15  N_points=1024  Kp=942.4778  Ki=222066.099  PositionUnit=Degrees  PositionDataType=single  FrequencyUnit=Degrees/Sec  FrequencyDataType=single  TableDataType=single
      settings: LibrarySourceBlock=mcblib/Signal Management/PLL with Feed Forward
  Sum : Sum  Inputs=|++
  ct : Outport
  Posdegree1 : Outport  Port=2  InitialOutput=0  VectorParamsAs1DForOutWhenUnconnected=off
  theta : Outport  Port=3  InitialOutput=0  VectorParamsAs1DForOutWhenUnconnected=off
  W : Outport  Port=4
  Halls : Outport  Port=5
  hallstate : Outport  Port=6
  wires:
  cti/1 -> ct/1
  Data Store Read7/1 -> Min/3
  Sum/1 -> Posdegree1/1
  Data Store Read6/1 -> hallstate/1, Discrete-Time Integrator/2, Hall Speed and Position1/6
  Hall Speed and Position1/2 -> Discrete-Time Integrator/1, W/1
  Data Store Read5/1 -> Hall Speed and Position1/5
  Hall Speed and Position1/1 -> Sum/1, theta/1
  Data Store Read1/1 -> Halls/1, Hall Speed and Position1/1
  Data Store Read2/1 -> Min/2
  Data Store Read4/1 -> Hall Speed and Position1/4
  Data Store Read3/1 -> Hall Speed and Position1/3
  Hall Speed and Position1/3 -> Data Store Write3/1
  Discrete-Time Integrator/1 -> Sum/2
  Data Store Read/1 -> Min/1
  Min/1 -> Hall Speed and Position1/2

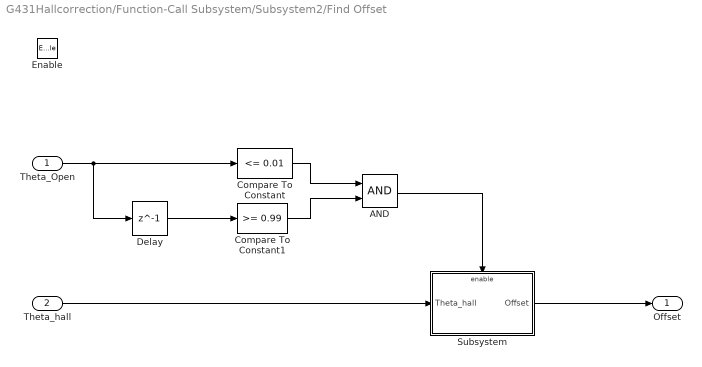
== system G431Hallcorrection/Function-Call Subsystem/Subsystem2/Find Offset ==
  Theta_Open : Inport
  Theta_hall : Inport  Port=2
  Enable : EnablePort  StatesWhenEnabling=reset
  AND : Logic  AllPortsSameDT=off  OutDataTypeStr=boolean
  Compare To Constant : simulink/Logic and Bit Operations/Compare To Constant  relop=<=  const=0.01  OutDataTypeStr=boolean
  Compare To Constant1 : simulink/Logic and Bit Operations/Compare To Constant  relop=>=  const=0.99  OutDataTypeStr=boolean
  Delay : Delay  DelayLength=1
  Subsystem : Subsystem
  Offset : Outport
  wires:
  Theta_Open/1 -> Delay/1, Compare To Constant/1
  Delay/1 -> Compare To Constant1/1
  Compare To Constant/1 -> AND/1
  Compare To Constant1/1 -> AND/2
  Theta_hall/1 -> Subsystem/1(Theta_hall)
  AND/1 -> Subsystem/Enable
  Subsystem/1(Offset) -> Offset/1

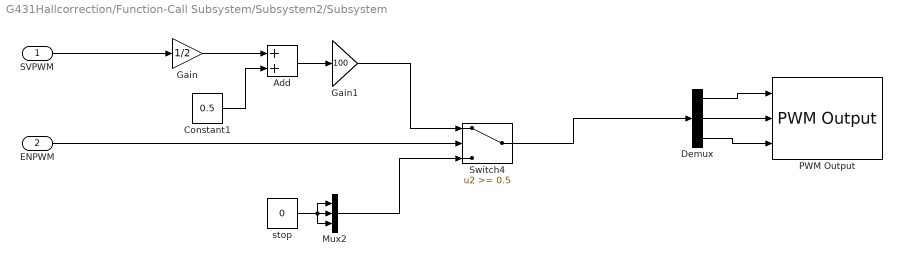
== system G431Hallcorrection/Function-Call Subsystem/Subsystem2/Subsystem ==
  SVPWM : Inport
  ENPWM : Inport  Port=2
  Add : Sum
  Constant1 : Constant  Value=0.5
  Demux : Demux  Outputs=3
  Gain : Gain  Gain=1/2
  Gain1 : Gain  Gain=100
  Mux2 : Mux  Inputs=3
  PWM Output : stm32g4xxblockslib/PWM Output  TimerModule=TIM1  DutycycleUnits=Percentage  EnableChannel1=on  EnableChannel2=on  EnableChannel3=on  EnableChannel4=off  EnableChannel5=off  EnableChannel6=off  EnableCounterInput=off  EnableMainOutputInput=off  EnableFrequencyInput=off  SetRCAfterCE=on  OutputDirection=off  OutputMainOutputEnableStatus=off  SampleTime=0.1  EnableSimPort=off  EnableUpdateEvent=off  EnableCaptureCompare1Event=off  EnableCaptureCompare2Event=off  EnableCaptureCompare3Event=off  EnableCaptureCompare4Event=off  EnableTriggerEvent=off  EnableBreakEvent=off  EnableBreakEvent2=off  ProcessorFamily=STM32G4  hoistedMaskSrc=ECSoC/ECSimCodegen/PWM Output
  Switch4 : Switch  Threshold=0.5  SaturateOnIntegerOverflow=off  InputSameDT=off
  stop : Constant  Value=0  OutDataTypeStr=uint16
  wires:
  Gain1/1 -> Switch4/1
  Gain/1 -> Add/1
  Add/1 -> Gain1/1
  ENPWM/1 -> Switch4/2
  stop/1 -> Mux2/2, Mux2/3, Mux2/1
  Constant1/1 -> Add/2
  SVPWM/1 -> Gain/1
  Switch4/1 -> Demux/1
  Mux2/1 -> Switch4/3
  Demux/2 -> PWM Output/2
  Demux/1 -> PWM Output/1
  Demux/3 -> PWM Output/3

== system G431Hallcorrection/Function-Call Subsystem/Subsystem2/Subsystem1 ==
  Input : Inport
  Enable : EnablePort
  Offset : Outport
  wires:
  Input/1 -> Offset/1

== system G431Hallcorrection/Function-Call Subsystem/Subsystem2/Subsystem2 ==
  sin : Inport
  cos : Inport  Port=2
  Inverse Park Transform : mcbcontrolslib/Inverse Park Transform  PhaseInput=Two inputs  AxisAlignment=D-axis  ThetaInput=Sine and Cosine electrical position  AngleInput=Per-unit  N_points=1024
  Mux : Mux  Inputs=3
  PWM Reference Generator : mcbcontrolslib/PWM Reference Generator  inSignal=Valphabeta  modType=SVM: space vector modulation
      settings: LibrarySourceBlock=mcblib/Controls/Math Transforms/PWM Reference Generator
  Vd_Ref : Constant  Value=0  VectorParams1D=off  OutMin=0  OutMax=1  OutDataTypeStr=single  SampleTime=-1
  Vq : Constant  Value=0.22  VectorParams1D=off  OutDataTypeStr=single  SampleTime=-1
  "SVPWM " : Outport
  wires:
  PWM Reference Generator/3 -> Mux/3
  PWM Reference Generator/2 -> Mux/2
  Vq/1 -> Inverse Park Transform/2
  Vd_Ref/1 -> Inverse Park Transform/1
  PWM Reference Generator/1 -> Mux/1
  cos/1 -> Inverse Park Transform/4
  Inverse Park Transform/1 -> PWM Reference Generator/1
  sin/1 -> Inverse Park Transform/3
  Inverse Park Transform/2 -> PWM Reference Generator/2
  Mux/1 -> "SVPWM "/1

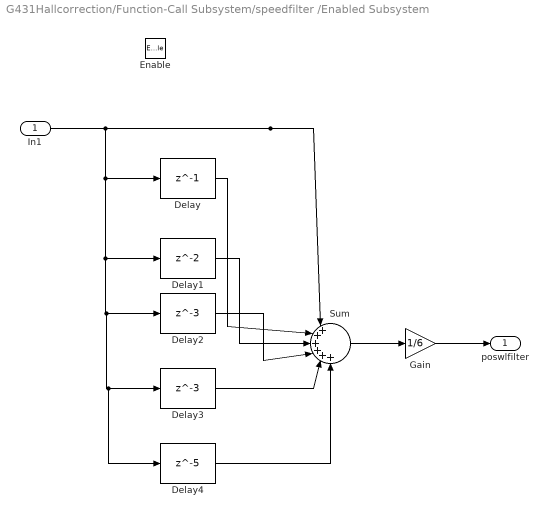
== system G431Hallcorrection/Function-Call Subsystem/speedfilter /Enabled Subsystem ==
  In1 : Inport
  Enable : EnablePort
  Delay : Delay  DelayLength=1  InitialCondition=0  UseCircularBuffer=on
  Delay1 : Delay
  Delay2 : Delay  DelayLength=3
  Delay3 : Delay  DelayLength=3
  Delay4 : Delay  DelayLength=5
  Gain : Gain  Gain=1/6
  Sum : Sum  Inputs=|++++++
  poswlfilter : Outport
  wires:
  In1/1 -> Delay4/1, Delay3/1, Delay2/1, Delay1/1, Delay/1, Sum/1
  Delay4/1 -> Sum/6
  Delay3/1 -> Sum/5
  Delay2/1 -> Sum/4
  Delay1/1 -> Sum/3
  Delay/1 -> Sum/2
  Sum/1 -> Gain/1
  Gain/1 -> poswlfilter/1

== system G431Hallcorrection/Function-Call Subsystem/Subsystem/PosGen/Subsystem ==
  Enable : EnablePort

== system G431Hallcorrection/Function-Call Subsystem/Subsystem/PosGen/Subsystem1 ==
  Count : Inport
  Count for 2 sec : Constant  Value=2.5 * 10000  OutDataTypeStr=uint32  SampleTime=-1
  If : If  NumInputs=2  IfExpression=u1 < u2
  If Action Subsystem : Subsystem  TreatAsAtomicUnit=on
  If Action Subsystem2 : Subsystem  TreatAsAtomicUnit=on
  Merge : Merge
  Position Generator : mcbcontrolslib/Position Generator  AngleOutput=Per-unit  ExternalReset=none  Offset=0
  Eps : Outport
  wires:
  If Action Subsystem/1(Out1) -> Merge/1
  If/1 -> If Action Subsystem/Action
  If Action Subsystem2/1(Out1) -> Merge/2
  Position Generator/1 -> Eps/1  "Eps"
  Count/1 -> If/1
  Merge/1 -> Position Generator/1
  If/2 -> If Action Subsystem2/Action
  Count for 2 sec/1 -> If/2

== system G431Hallcorrection/Function-Call Subsystem/Subsystem/PosGen/Up Counter ==
  Enable : EnablePort  StatesWhenEnabling=reset
  Add1 : Sum  SaturateOnIntegerOverflow=on
  Constant : Constant  OutDataTypeStr=uint32
  Delay : Delay  DelayLength=1
  Count : Outport  OutputWhenDisabled=reset  InitialOutput=0
  wires:
  Add1/1 -> Count/1, Delay/1
  Constant/1 -> Add1/1
  Delay/1 -> Add1/2

== system G431Hallcorrection/Function-Call Subsystem/Subsystem2/Find Offset/Subsystem ==
  Theta_hall : Inport
  Enable : EnablePort
  IIR Filter : mcbcontrolslib/IIR Filter  VariantControl=Low Pass Filter  VariantSelect=Low-pass  FilterConstantInputType=Specify via dialog  Filter_constant=0.5  advancedSettings=off  Ts=50e-6  cutOff_freq=3183.0989
  Offset : Outport
  wires:
  IIR Filter/1 -> Offset/1
  Theta_hall/1 -> IIR Filter/1

== system G431Hallcorrection/Function-Call Subsystem/Subsystem/PosGen/Subsystem1/If Action Subsystem ==
  Action Port : ActionPort  ActionPortLabel=if(u1 < u2)
  Constant : Constant  Value=0  OutDataTypeStr=single
  Out1 : Outport
  wires:
  Constant/1 -> Out1/1

== system G431Hallcorrection/Function-Call Subsystem/Subsystem/PosGen/Subsystem1/If Action Subsystem2 ==
  Action Port : ActionPort  ActionPortLabel=else
  Add1 : Sum
  Constant1 : Constant  Value=2e-4  VectorParams1D=off  OutDataTypeStr=single
  Delay : Delay  DelayLength=1
  Multiply : Gain  Gain=1e-4  OutDataTypeStr=Inherit: Same as input
  Saturate to 'motor.calibSpeed' RPM : Saturate  UpperLimit=2 *240/ 60  LowerLimit=0
  Out1 : Outport
  wires:
  Delay/1 -> Add1/2
  Constant1/1 -> Add1/1
  Multiply/1 -> Out1/1
  Add1/1 -> Saturate to 'motor.calibSpeed' RPM/1
  Saturate to 'motor.calibSpeed' RPM/1 -> Delay/1, Multiply/1
